simulink model "Anfis_sist_no_lineal_validacion"  (R2016a)
settings: Solver=VariableStepAuto  StartTime=0.0  StopTime=200  RelTol=1e-3
values from neighbouring files (symbols this model uses):
  b = [1;1]    [ejemplodiscretro.m]
undefined symbols (not defined in the file or in its folder): Anfis_sist_no_lineal_blok, k
libraries: fuzblock x1
settings Model: Creator=Daniel  LastModifiedBy=Daniel

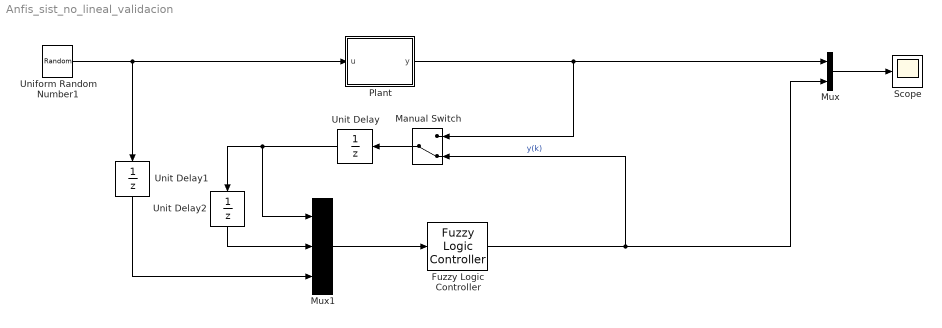
== system Anfis_sist_no_lineal_validacion ==
  Fuzzy Logic Controller : fuzblock/Fuzzy Logic  Controller  fis=[Anfis_sist_no_lineal_blok]
  Manual Switch : ManualSwitch  CurrentSetting=0
  Mux : Mux  Inputs=2
  Mux1 : Mux  Inputs=3
  Plant : Subsystem
  Scope : Scope
  Uniform Random Number1 : UniformRandomNumber  Minimum=0  Maximum=5  SampleTime=10
  Unit Delay : UnitDelay  SampleTime=0.1
  Unit Delay1 : UnitDelay  SampleTime=0.1
  Unit Delay2 : UnitDelay  SampleTime=0.1
  wires:
  Uniform Random Number1/1 -> Plant/1(u), Unit Delay1/1
  Fuzzy Logic Controller/1 -> Manual Switch/2, Mux/2  "y(k)"
  Manual Switch/1 -> Unit Delay/1
  Unit Delay/1 -> Mux1/1, Unit Delay2/1
  Mux/1 -> Scope/1
  Mux1/1 -> Fuzzy Logic Controller/1
  Plant/1(y) -> Manual Switch/1, Mux/1
  Unit Delay2/1 -> Mux1/2
  Unit Delay1/1 -> Mux1/3

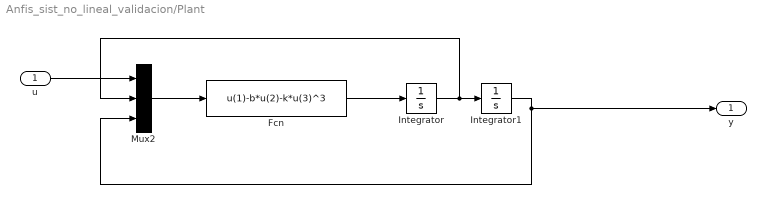
== system Anfis_sist_no_lineal_validacion/Plant ==
  u : Inport
  Fcn : Fcn  Expr=u(1)-b*u(2)-k*u(3)^3
  Integrator : Integrator
  Integrator1 : Integrator
  Mux2 : Mux  Inputs=3
  y : Outport
  wires:
  Fcn/1 -> Integrator/1
  Integrator/1 -> Mux2/2, Integrator1/1
  Integrator1/1 -> y/1, Mux2/3
  Mux2/1 -> Fcn/1
  u/1 -> Mux2/1
